simulink library "enginelib"  (Simulink 7.2)
settings: Solver=ode45  SolverMode=SingleTasking  StartTime=0.0  StopTime=10.0  RelTol=1e-3
libraries: engine_T2_lib x3, engine_JetCatP70_lib x2, engine_AMT180_lib x1, engine_AMT280_lib x1, enginelib x1, engine_JetCatP120SE_lib x1, simulink x1
settings Model: Creator=cox  LastModifiedBy=E183308  ExtModeAutoUpdateStatusClock=off

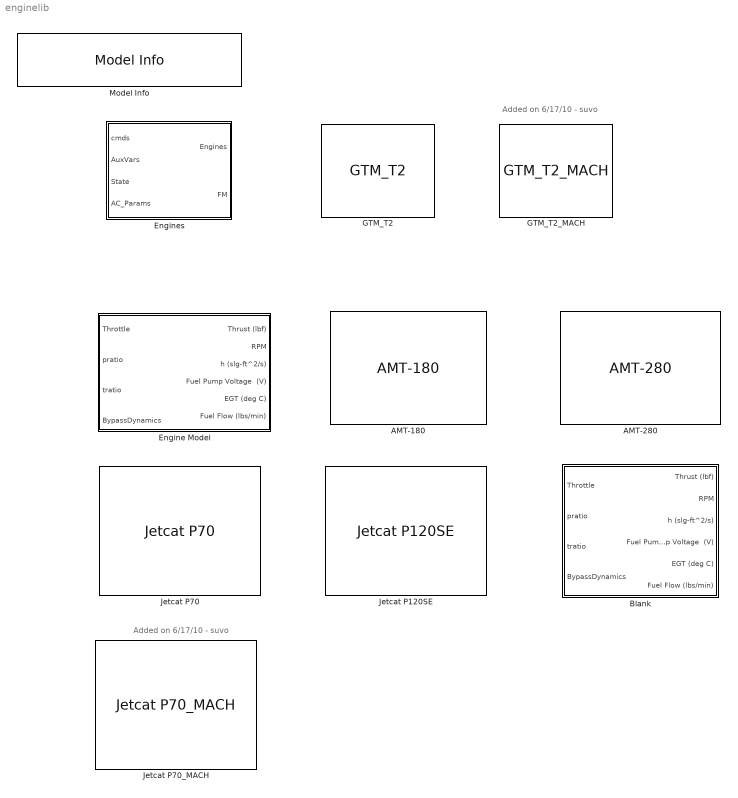
== system enginelib ==
  note: Added on 6/17/10 - suvo
  note: Added on 6/17/10 - suvo
  AMT-180 : engine_AMT180_lib/AMT-180  SystemSampleTime=-1
  AMT-280 : engine_AMT280_lib/AMT-280  SystemSampleTime=-1
  Blank : Subsystem
      mask init:
      | % Curve fit parameters for AMT-280 Model
      | Coeff_thrust   = [ 5.7372e-05  -5.2629e-03   3.1586e-01  -5.1517e+00];
      | Coeff_throttle = [ -4.3078e-03   1.1110e+00   2.9012e+01];
      | Coeff_fuelflow = [ 1.0140e-04  -1.5867e-03   2.0125e-01];
      | Coeff_tau      = [ -2.2400e-02   2.9948e+00];
      | 
      | 
      | % Equvalent Shaft parameters for engine
      | shaft_dia = 0.75/12.0;       % diameter of rotating turbine in feet 
      | shaft_len = 6.25/12.0;       % length of rotating turbine in feet   
      | density   = 15.2;            % mass density of steel in slugs/ft^3
  Engine Model : Subsystem  BlockChoice=Blank
      settings: TemplateBlock=self  MemberBlocks=AMT-180,AMT-280,Blank,Jetcat P120SE,Jetcat P70,Jetcat P70_MACH
  Engines : Subsystem  BlockChoice=GTM_T2
      settings: TemplateBlock=self  MemberBlocks=GTM_T2,GTM_T2_MACH
  GTM_T2 : engine_T2_lib/GTM_T2  SystemSampleTime=-1
  GTM_T2_MACH : engine_T2_lib/GTM_T2_MACH  SystemSampleTime=-1
  Jetcat P120SE : engine_JetCatP120SE_lib/Jetcat P120SE  SystemSampleTime=-1
  Jetcat P70 : engine_JetCatP70_lib/Jetcat P70  SystemSampleTime=-1
  Jetcat P70_MACH : engine_JetCatP70_lib/Jetcat P70_MACH  SystemSampleTime=-1
  Model Info : simulink/Model-Wide Utilities/Model Info  SystemSampleTime=-1  InitialBlockCM=none  BlockCM=none  Frame=on  DisplayStringWithTags=|  HorizontalTextAlignment=Center  LeftAlignmentValue=0.5  SourceBlockDiagram=enginelib  TagMaxNumber=20
      | engine library
      | 
      | Model Version: %<ModelVersion>
      | Last modifed by %<LastModifiedBy> on %<LastModificationDate>

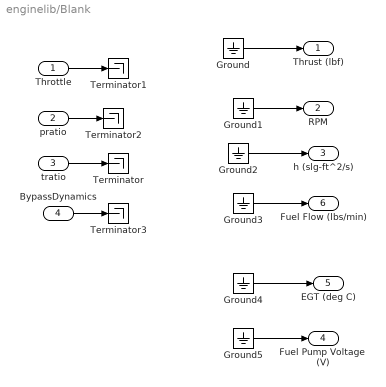
== system enginelib/Blank ==
  Throttle : Inport  OutDataType=sfix(16)  OutScaling=2^0
  pratio : Inport  Port=2  OutDataType=sfix(16)  OutScaling=2^0
  tratio : Inport  Port=3  OutDataType=sfix(16)  OutScaling=2^0
  BypassDynamics : Inport  Port=4  OutDataType=sfix(16)  OutScaling=2^0
  Ground{,1..5} (6 alike) : Ground
  Terminator{,1..3} (4 alike) : Terminator
  Thrust (lbf) : Outport  OutDataType=sfix(16)  OutScaling=2^0
  RPM : Outport  Port=2  OutDataType=sfix(16)  OutScaling=2^0
  h (slg-ft^2/s) : Outport  Port=3  OutDataType=sfix(16)  OutScaling=2^0
  Fuel Pump Voltage  (V) : Outport  Port=4  OutDataType=sfix(16)  OutScaling=2^0
  EGT (deg C) : Outport  Port=5  OutDataType=sfix(16)  OutScaling=2^0
  Fuel Flow (lbs/min) : Outport  Port=6  OutDataType=sfix(16)  OutScaling=2^0
  wires:
  Throttle/1 -> Terminator1/1
  pratio/1 -> Terminator2/1
  tratio/1 -> Terminator/1
  Ground/1 -> Thrust (lbf)/1
  Ground1/1 -> RPM/1
  Ground2/1 -> h (slg-ft^2/s)/1
  Ground5/1 -> Fuel Pump Voltage  (V)/1
  Ground4/1 -> EGT (deg C)/1
  Ground3/1 -> Fuel Flow (lbs/min)/1
  BypassDynamics/1 -> Terminator3/1

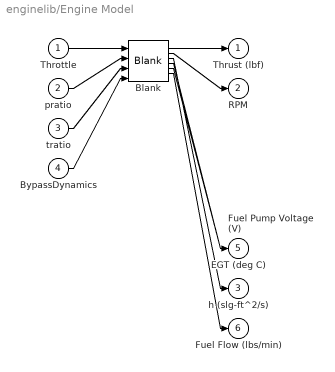
== system enginelib/Engine Model ==
  Throttle : Inport  OutDataType=sfix(16)  OutScaling=2^0
  pratio : Inport  Port=2  OutDataType=sfix(16)  OutScaling=2^0
  tratio : Inport  Port=3  OutDataType=sfix(16)  OutScaling=2^0
  BypassDynamics : Inport  Port=4  OutDataType=sfix(16)  OutScaling=2^0
  Blank : enginelib/Blank  SystemSampleTime=-1
  Thrust (lbf) : Outport  OutDataType=sfix(16)  OutScaling=2^0
  RPM : Outport  Port=2  OutDataType=sfix(16)  OutScaling=2^0
  h (slg-ft^2/s) : Outport  Port=3  OutDataType=sfix(16)  OutScaling=2^0
  Fuel Pump Voltage  (V) : Outport  Port=4  OutDataType=sfix(16)  OutScaling=2^0
  EGT (deg C) : Outport  Port=5  OutDataType=sfix(16)  OutScaling=2^0
  Fuel Flow (lbs/min) : Outport  Port=6  OutDataType=sfix(16)  OutScaling=2^0
  wires:
  Throttle/1 -> Blank/1
  pratio/1 -> Blank/2
  tratio/1 -> Blank/3
  BypassDynamics/1 -> Blank/4
  Blank/1 -> Thrust (lbf)/1
  Blank/2 -> RPM/1
  Blank/3 -> h (slg-ft^2/s)/1
  Blank/4 -> Fuel Pump Voltage  (V)/1
  Blank/5 -> EGT (deg C)/1
  Blank/6 -> Fuel Flow (lbs/min)/1

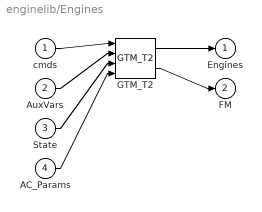
== system enginelib/Engines ==
  cmds : Inport  OutDataType=sfix(16)  OutScaling=2^0
  AuxVars : Inport  Port=2  OutDataType=sfix(16)  OutScaling=2^0
  State : Inport  Port=3  OutDataType=sfix(16)  OutScaling=2^0
  AC_Params : Inport  Port=4  OutDataType=sfix(16)  OutScaling=2^0
  GTM_T2 : engine_T2_lib/GTM_T2  SystemSampleTime=-1
  Engines : Outport  OutDataType=sfix(16)  OutScaling=2^0
  FM : Outport  Port=2  OutDataType=sfix(16)  OutScaling=2^0
  wires:
  cmds/1 -> GTM_T2/1
  AuxVars/1 -> GTM_T2/2
  State/1 -> GTM_T2/3
  AC_Params/1 -> GTM_T2/4
  GTM_T2/1 -> Engines/1
  GTM_T2/2 -> FM/1
